simulink model "omnibundle_descentr_joint"  (R2018b)
settings: Solver=ode23t  StartTime=0.0  StopTime=9  FixedStep=0.01  RelTol=1e-3
values from neighbouring files (symbols this model uses):
  ddqv = ddt(ddt(qv,dt),dt)    [main.m]    (also in traj_planning.m = ddt(ddt(qv,dts),dts))
  dq0 = [0 0 0]'    [main.m]
  dqv = ddt(qv,dt)    [main.m]    (also in traj_planning.m = ddt(qv,dts))
  Km = inv(fv)    [main.m]
  Kp = wn^2./diag(Km)./Kv    [main.m]
  Kv = 2*zeta*wn./diag(Km)    [main.m]
  q0 = qs(1,2:4)'    [main.m]
  qv = []    [main.m]    (also in traj_planning.m)
  tv = 0:dt:qs(end,1)    [main.m]    (also in traj_planning.m = 0:dts:qs(end,1))
  Tv = diag(Tm)    [main.m]
libraries: simulink x3
settings Model: Creator=Renata  LastModifiedBy=lucas

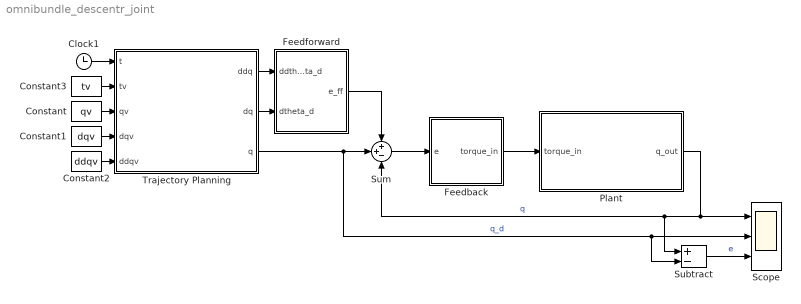
== system omnibundle_descentr_joint ==
  Clock1 : Clock
  Constant : Constant  Value=qv
  Constant1 : Constant  Value=dqv
  Constant2 : Constant  Value=ddqv
  Constant3 : Constant  Value=tv
  Feedback : Subsystem
  Feedforward : Subsystem
  Plant : Subsystem
  Scope : Scope  NumInputPorts=3
  Subtract : Sum  Inputs=+-
  Sum : Sum  Inputs=++-
  Trajectory Planning : MATLAB Function  TreatAsAtomicUnit=on
  wires:
  Feedback/1(torque_in) -> Plant/1(torque_in)
  Plant/1(q_out) -> Subtract/1, Sum/3, Scope/1  "q"
  Sum/1 -> Feedback/1(e)
  Feedforward/1(e_ff) -> Sum/1
  Trajectory Planning/1(ddq) -> Feedforward/1(ddtheta_d)
  Trajectory Planning/2(dq) -> Feedforward/2(dtheta_d)
  Trajectory Planning/3(q) -> Subtract/2, Scope/2, Sum/2  "q_d"
  Subtract/1 -> Scope/3  "e"
  Clock1/1 -> Trajectory Planning/1(t)
  Constant/1 -> Trajectory Planning/3(qv)
  Constant2/1 -> Trajectory Planning/5(ddqv)
  Constant1/1 -> Trajectory Planning/4(dqv)
  Constant3/1 -> Trajectory Planning/2(tv)

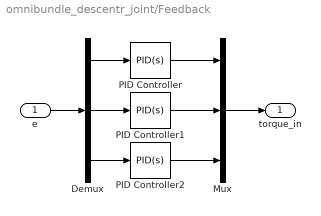
== system omnibundle_descentr_joint/Feedback ==
  e : Inport
  Demux : Demux  Outputs=3
  Mux : Mux  Inputs=3
  PID Controller : simulink/Continuous/PID Controller  Controller=PID  Form=Parallel  TimeDomain=Continuous-time  SampleTime=-1  IntegratorMethod=Forward Euler  FilterMethod=Forward Euler  ControllerParametersSource=internal  P=Kv(1)+Kp(1)*Kv(1)*Tv(1)  I=Kp(1)*Kv(1)  D=Kv(1)*Tv(1)  UseFilter=on  N=1000  TunerSelectOption=Transfer Function Based (PID Tuner App)  ZeroCross=off  InitialConditionSource=internal  InitialConditionForIntegrator=0  InitialConditionForFilter=0  DifferentiatorICPrevScaledInput=0  ExternalReset=none  TrackingMode=off  Kt=1  LimitOutput=off  UpperSaturationLimit=inf  LowerSaturationLimit=-inf  LinearizeAsGain=on  AntiWindupMode=none  Kb=1  POutMin=[]  POutMax=[]  IOutMin=[]  IOutMax=[]  DOutMin=[]  DOutMax=[]  NOutMin=[]  NOutMax=[]  SumOutMin=[]  SumOutMax=[]  SaturationOutMin=[]  SaturationOutMax=[]  PParamMin=[]  PParamMax=[]  IParamMin=[]  IParamMax=[]  DParamMin=[]  DParamMax=[]  NParamMin=[]  NParamMax=[]  KbParamMin=[]  KbParamMax=[]  KtParamMin=[]  KtParamMax=[]  KbOutMin=[]  KbOutMax=[]  KtOutMin=[]  KtOutMax=[]  IntegratorOutMin=[]  IntegratorOutMax=[]  FilterOutMin=[]  FilterOutMax=[]  SumI1OutMin=[]  SumI1OutMax=[]  SumI2OutMin=[]  SumI2OutMax=[]  SumI3OutMin=[]  SumI3OutMax=[]  SumI4OutMin=[]  SumI4OutMax=[]  SumDOutMin=[]  SumDOutMax=[]  DifferentiatorOutMin=[]  DifferentiatorOutMax=[]  FilterDiffOutCoefMin=[]  FilterDiffOutCoefMax=[]  ReciprocalOutMin=[]  ReciprocalOutMax=[]  SumDenOutMin=[]  SumDenOutMax=[]  SumNumOutMin=[]  SumNumOutMax=[]  DivideOutMin=[]  DivideOutMax=[]  IntegratorContinuousStateAttributes=''  IntegratorStateMustResolveToSignalObject=off  IntegratorRTWStateStorageClass=Auto  FilterContinuousStateAttributes=''  FilterStateMustResolveToSignalObject=off  FilterRTWStateStorageClass=Auto  ParallelPVariant=InternalParameters  IdealPVariant=Disabled  IVariant=InternalParameters  DVariant=InternalParameters  IntegratorVariant=Continuous  SatVariant=Disabled  AWVariant=Passthrough  PCopyVariant=Disabled  TRVariant=Disabled  FdbkBlocksVariant=Forward  IdealPFdbkVariant=Disabled  SatFdbkVariant=Disabled  DerivativeFilterVariant=ContFilter  NVariant=InternalParameters  NCopyVariant=Disabled  FilterICVariant=InternalICsFilter  IntegratorICVariant=InternalICs  ExternalResetVariant=Disabled  TRSumVariant=Passthrough  SumFdbkVariant=Disabled  SumVariant=Sum_PID
  PID Controller1 : simulink/Continuous/PID Controller  Controller=PID  Form=Parallel  TimeDomain=Continuous-time  SampleTime=-1  IntegratorMethod=Forward Euler  FilterMethod=Forward Euler  ControllerParametersSource=internal  P=Kv(2)+Kp(2)*Kv(2)*Tv(2)  I=Kp(2)*Kv(2)  D=Kv(2)*Tv(2)  UseFilter=on  N=1000  TunerSelectOption=Transfer Function Based (PID Tuner App)  ZeroCross=off  InitialConditionSource=internal  InitialConditionForIntegrator=0  InitialConditionForFilter=0  DifferentiatorICPrevScaledInput=0  ExternalReset=none  TrackingMode=off  Kt=1  LimitOutput=off  UpperSaturationLimit=inf  LowerSaturationLimit=-inf  LinearizeAsGain=on  AntiWindupMode=none  Kb=1  POutMin=[]  POutMax=[]  IOutMin=[]  IOutMax=[]  DOutMin=[]  DOutMax=[]  NOutMin=[]  NOutMax=[]  SumOutMin=[]  SumOutMax=[]  SaturationOutMin=[]  SaturationOutMax=[]  PParamMin=[]  PParamMax=[]  IParamMin=[]  IParamMax=[]  DParamMin=[]  DParamMax=[]  NParamMin=[]  NParamMax=[]  KbParamMin=[]  KbParamMax=[]  KtParamMin=[]  KtParamMax=[]  KbOutMin=[]  KbOutMax=[]  KtOutMin=[]  KtOutMax=[]  IntegratorOutMin=[]  IntegratorOutMax=[]  FilterOutMin=[]  FilterOutMax=[]  SumI1OutMin=[]  SumI1OutMax=[]  SumI2OutMin=[]  SumI2OutMax=[]  SumI3OutMin=[]  SumI3OutMax=[]  SumI4OutMin=[]  SumI4OutMax=[]  SumDOutMin=[]  SumDOutMax=[]  DifferentiatorOutMin=[]  DifferentiatorOutMax=[]  FilterDiffOutCoefMin=[]  FilterDiffOutCoefMax=[]  ReciprocalOutMin=[]  ReciprocalOutMax=[]  SumDenOutMin=[]  SumDenOutMax=[]  SumNumOutMin=[]  SumNumOutMax=[]  DivideOutMin=[]  DivideOutMax=[]  IntegratorContinuousStateAttributes=''  IntegratorStateMustResolveToSignalObject=off  IntegratorRTWStateStorageClass=Auto  FilterContinuousStateAttributes=''  FilterStateMustResolveToSignalObject=off  FilterRTWStateStorageClass=Auto  ParallelPVariant=InternalParameters  IdealPVariant=Disabled  IVariant=InternalParameters  DVariant=InternalParameters  IntegratorVariant=Continuous  SatVariant=Disabled  AWVariant=Passthrough  PCopyVariant=Disabled  TRVariant=Disabled  FdbkBlocksVariant=Forward  IdealPFdbkVariant=Disabled  SatFdbkVariant=Disabled  DerivativeFilterVariant=ContFilter  NVariant=InternalParameters  NCopyVariant=Disabled  FilterICVariant=InternalICsFilter  IntegratorICVariant=InternalICs  ExternalResetVariant=Disabled  TRSumVariant=Passthrough  SumFdbkVariant=Disabled  SumVariant=Sum_PID
  PID Controller2 : simulink/Continuous/PID Controller  Controller=PID  Form=Parallel  TimeDomain=Continuous-time  SampleTime=-1  IntegratorMethod=Forward Euler  FilterMethod=Forward Euler  ControllerParametersSource=internal  P=Kv(3)+Kp(3)*Kv(3)*Tv(3)  I=Kp(3)*Kv(3)  D=Kv(3)*Tv(3)  UseFilter=on  N=1000  TunerSelectOption=Transfer Function Based (PID Tuner App)  ZeroCross=off  InitialConditionSource=internal  InitialConditionForIntegrator=0  InitialConditionForFilter=0  DifferentiatorICPrevScaledInput=0  ExternalReset=none  TrackingMode=off  Kt=1  LimitOutput=off  UpperSaturationLimit=inf  LowerSaturationLimit=-inf  LinearizeAsGain=on  AntiWindupMode=none  Kb=1  POutMin=[]  POutMax=[]  IOutMin=[]  IOutMax=[]  DOutMin=[]  DOutMax=[]  NOutMin=[]  NOutMax=[]  SumOutMin=[]  SumOutMax=[]  SaturationOutMin=[]  SaturationOutMax=[]  PParamMin=[]  PParamMax=[]  IParamMin=[]  IParamMax=[]  DParamMin=[]  DParamMax=[]  NParamMin=[]  NParamMax=[]  KbParamMin=[]  KbParamMax=[]  KtParamMin=[]  KtParamMax=[]  KbOutMin=[]  KbOutMax=[]  KtOutMin=[]  KtOutMax=[]  IntegratorOutMin=[]  IntegratorOutMax=[]  FilterOutMin=[]  FilterOutMax=[]  SumI1OutMin=[]  SumI1OutMax=[]  SumI2OutMin=[]  SumI2OutMax=[]  SumI3OutMin=[]  SumI3OutMax=[]  SumI4OutMin=[]  SumI4OutMax=[]  SumDOutMin=[]  SumDOutMax=[]  DifferentiatorOutMin=[]  DifferentiatorOutMax=[]  FilterDiffOutCoefMin=[]  FilterDiffOutCoefMax=[]  ReciprocalOutMin=[]  ReciprocalOutMax=[]  SumDenOutMin=[]  SumDenOutMax=[]  SumNumOutMin=[]  SumNumOutMax=[]  DivideOutMin=[]  DivideOutMax=[]  IntegratorContinuousStateAttributes=''  IntegratorStateMustResolveToSignalObject=off  IntegratorRTWStateStorageClass=Auto  FilterContinuousStateAttributes=''  FilterStateMustResolveToSignalObject=off  FilterRTWStateStorageClass=Auto  ParallelPVariant=InternalParameters  IdealPVariant=Disabled  IVariant=InternalParameters  DVariant=InternalParameters  IntegratorVariant=Continuous  SatVariant=Disabled  AWVariant=Passthrough  PCopyVariant=Disabled  TRVariant=Disabled  FdbkBlocksVariant=Forward  IdealPFdbkVariant=Disabled  SatFdbkVariant=Disabled  DerivativeFilterVariant=ContFilter  NVariant=InternalParameters  NCopyVariant=Disabled  FilterICVariant=InternalICsFilter  IntegratorICVariant=InternalICs  ExternalResetVariant=Disabled  TRSumVariant=Passthrough  SumFdbkVariant=Disabled  SumVariant=Sum_PID
  torque_in : Outport
  wires:
  Mux/1 -> torque_in/1
  e/1 -> Demux/1
  Demux/1 -> PID Controller/1
  PID Controller/1 -> Mux/1
  Demux/3 -> PID Controller2/1
  PID Controller2/1 -> Mux/3
  Demux/2 -> PID Controller1/1
  PID Controller1/1 -> Mux/2

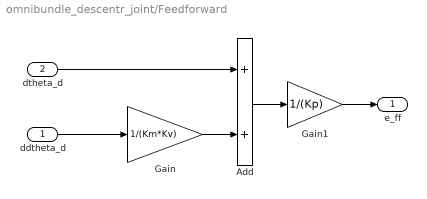
== system omnibundle_descentr_joint/Feedforward ==
  ddtheta_d : Inport
  dtheta_d : Inport  Port=2
  Add : Sum
  Gain : Gain  Gain=1/(Km*Kv)
  Gain1 : Gain  Gain=1/(Kp)
  e_ff : Outport
  wires:
  Add/1 -> Gain1/1
  dtheta_d/1 -> Add/1
  ddtheta_d/1 -> Gain/1
  Gain/1 -> Add/2
  Gain1/1 -> e_ff/1

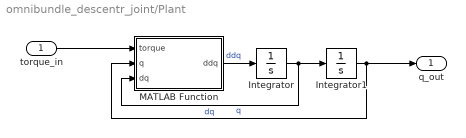
== system omnibundle_descentr_joint/Plant ==
  torque_in : Inport
  Integrator : Integrator  InitialCondition=dq0
  Integrator1 : Integrator  InitialCondition=q0
  MATLAB Function : MATLAB Function  TreatAsAtomicUnit=on
  q_out : Outport
  wires:
  MATLAB Function/1(ddq) -> Integrator/1  "ddq"
  Integrator/1 -> MATLAB Function/3(dq), Integrator1/1  "dq"
  torque_in/1 -> MATLAB Function/1(torque)
  Integrator1/1 -> q_out/1, MATLAB Function/2(q)  "q"

== matlab function omnibundle_descentr_joint/Plant/MATLAB Function ==
  data: torque input; q input; dq input; ddq output
function ddq = fcn(torque,q,dq)
    
    ddq = dyn_omni_bundle_fun(9.8, q, dq, torque);

== matlab function omnibundle_descentr_joint/Trajectory Planning ==
  data: t input; tv input; ddq output; dq output; q output; qv input; dqv input; ddqv input
function [ddq,dq,q] = trajectory_planning(t, tv, qv, dqv, ddqv)

    if t > tv(end-2)
        t = tv(end-2);
    end

    q = interp1(tv',qv',t)';
    dq = interp1(tv(1:end-1)',dqv',t)';
    ddq = interp1(tv(1:end-2)',ddqv',t)';
